simulink model "gap_generation_single_veh_state_machine"  (R2019a)
settings: Solver=VariableStepAuto  StartTime=0.0  StopTime=40  FixedStep=0.1  RelTol=1e-3
undefined symbols (not defined in the file): DiscIntNeverNeededParam
libraries: simulink x43, powerlib_meascontrol x5, autolibshared x5
(part 3 of 3)

== system gap_generation_single_veh_state_machine/Lo/ACC/Headway error ==
  xf : Inport
  vf : Inport  Port=2
  xl : Inport  Port=3
  lcFlag : Inport  Port=4
  Compare To Constant : simulink/Logic and Bit Operations/Compare To Constant  relop=<=  const=0  OutDataTypeStr=boolean
  Demux{,1..3} (4 alike) : Demux  Outputs=2
  Integrator : Integrator  InitialCondition=[h d0]
  Multiply : Product
  Mux : Mux  Inputs=2
  Mux1 : Mux  Inputs=2
  Product : Product
  Sum : Sum  Inputs=-+|
  Sum1 : Sum  Inputs=++|
  Sum2 : Sum  Inputs=+-|
  Sum3 : Sum  Inputs=|++
  Sum4 : Sum  Inputs=|+-
  Sum5 : Sum  Inputs=+-|
  Sum6 : Sum  Inputs=|++
  Switch : Switch  Criteria=u2 > Threshold
  Terminator : Terminator
  Terminator1 : Terminator
  d0 : Constant  Value=d0
  d0Lc : Constant  Value=d0Lc
  h : Constant  Value=h
  h scope : Scope  NumInputPorts=2
  hFilterGain : Gain  Gain=hFilterGain
  hLc : Constant  Value=hLc
  vLen : Constant  Value=lr+lf
  eh : Outport
  "gap " : Outport  Port=2
  unsafeFlag : Outport  Port=3
  wires:
  Demux3/2 -> Terminator1/1
  Demux2/2 -> Terminator/1
  Demux3/1 -> h scope/2
  Demux2/1 -> h scope/1
  Sum6/1 -> Sum5/2  "safe  gap"
  Demux1/2 -> Sum6/2  "gap at  standstill"
  Product/1 -> Sum6/1
  Demux1/1 -> Product/2  "time headway"
  Compare To Constant/1 -> unsafeFlag/1
  Sum5/1 -> Compare To Constant/1
  hFilterGain/1 -> Integrator/1
  Demux/2 -> Sum3/2  "gap at  standstill"
  Demux/1 -> Multiply/2  "time headway"
  Mux1/1 -> Switch/1
  d0Lc/1 -> Mux1/2
  hLc/1 -> Mux1/1
  Mux/1 -> Switch/3, Demux1/1  "min safe gap"
  d0/1 -> Mux/2
  Sum2/1 -> eh/1
  lcFlag/1 -> Switch/2
  Integrator/1 -> Demux/1, Sum4/2, Demux3/1
  Sum4/1 -> hFilterGain/1
  Switch/1 -> Sum4/1, Demux2/1
  h/1 -> Mux/1
  xl/1 -> Sum/2
  Sum1/1 -> Sum/1  "x (front bumber)"
  vf/1 -> Multiply/1, Product/1
  Sum3/1 -> Sum2/2  "desired  gap"
  xf/1 -> Sum1/2
  Sum/1 -> Sum2/1, "gap "/1, Sum5/1  "gap"
  Multiply/1 -> Sum3/1
  vLen/1 -> Sum1/1

== system gap_generation_single_veh_state_machine/Lo/ACC-v/Headway error ==
  xf : Inport
  vf : Inport  Port=2
  xl : Inport  Port=3
  lcFlag : Inport  Port=4
  Demux : Demux  Outputs=2
  Integrator : Integrator  InitialCondition=h
  Multiply : Product
  Mux : Mux  Inputs=2
  Mux1 : Mux  Inputs=2
  Sum : Sum  Inputs=-+|
  Sum1 : Sum  Inputs=++|
  Sum2 : Sum  Inputs=+-|
  Sum3 : Sum  Inputs=|++
  Sum4 : Sum  Inputs=|+-
  Switch : Switch  Criteria=u2 > Threshold
  d0 : Constant  Value=d0
  d0Lc : Constant  Value=d0Lc
  h : Constant  Value=h
  hFilterGain : Gain  Gain=hFilterGain
  hLc : Constant  Value=hLc
  vLen : Constant  Value=lr+lf
  eh : Outport
  "gap " : Outport  Port=2
  wires:
  Demux/2 -> Sum3/2  "gap at  standstill"
  Demux/1 -> Multiply/2  "time headway"
  Mux1/1 -> Switch/1
  d0Lc/1 -> Mux1/2
  hLc/1 -> Mux1/1
  Mux/1 -> Switch/3
  d0/1 -> Mux/2
  Sum2/1 -> eh/1
  lcFlag/1 -> Switch/2
  Integrator/1 -> Demux/1, Sum4/2
  Sum4/1 -> hFilterGain/1
  hFilterGain/1 -> Integrator/1
  Switch/1 -> Sum4/1
  h/1 -> Mux/1
  xl/1 -> Sum/2
  Sum1/1 -> Sum/1  "x (front bumber)"
  vf/1 -> Multiply/1
  Sum3/1 -> Sum2/2  "desired  gap"
  xf/1 -> Sum1/2
  Sum/1 -> Sum2/1, "gap "/1  "gap"
  Multiply/1 -> Sum3/1
  vLen/1 -> Sum1/1

== system gap_generation_single_veh_state_machine/Lo/ACC-v/Triggered Subsystem ==
  Trigger : TriggerPort  VariantControl=Variant
  Constant : Constant
  Out1 : Outport  InitialOutput=0
  wires:
  Constant/1 -> Out1/1

== system gap_generation_single_veh_state_machine/Lo/ACC-v/Triggered Subsystem1 ==
  Trigger : TriggerPort  VariantControl=Variant
  Constant : Constant  Value=0
  Out1 : Outport  InitialOutput=1
  wires:
  Constant/1 -> Out1/1

== system gap_generation_single_veh_state_machine/p1/ACC/Headway error ==
  xf : Inport
  vf : Inport  Port=2
  xl : Inport  Port=3
  lcFlag : Inport  Port=4
  Compare To Constant : simulink/Logic and Bit Operations/Compare To Constant  relop=<=  const=0  OutDataTypeStr=boolean
  Demux{,1..3} (4 alike) : Demux  Outputs=2
  Integrator : Integrator  InitialCondition=[h d0]
  Multiply : Product
  Mux : Mux  Inputs=2
  Mux1 : Mux  Inputs=2
  Product : Product
  Sum : Sum  Inputs=-+|
  Sum1 : Sum  Inputs=++|
  Sum2 : Sum  Inputs=+-|
  Sum3 : Sum  Inputs=|++
  Sum4 : Sum  Inputs=|+-
  Sum5 : Sum  Inputs=+-|
  Sum6 : Sum  Inputs=|++
  Switch : Switch  Criteria=u2 > Threshold
  Terminator : Terminator
  Terminator1 : Terminator
  d0 : Constant  Value=d0
  d0Lc : Constant  Value=d0Lc
  h : Constant  Value=h
  h scope : Scope  NumInputPorts=2
  hFilterGain : Gain  Gain=hFilterGain
  hLc : Constant  Value=hLc
  vLen : Constant  Value=lr+lf
  eh : Outport
  "gap " : Outport  Port=2
  unsafeFlag : Outport  Port=3
  wires:
  vLen/1 -> Sum1/1
  Multiply/1 -> Sum3/1
  Sum/1 -> Sum5/1, "gap "/1, Sum2/1  "gap"
  xf/1 -> Sum1/2
  Sum3/1 -> Sum2/2  "desired  gap"
  vf/1 -> Product/1, Multiply/1
  Sum1/1 -> Sum/1  "x (front bumber)"
  xl/1 -> Sum/2
  h/1 -> Mux/1
  Switch/1 -> Demux2/1, Sum4/1
  Sum4/1 -> hFilterGain/1
  Integrator/1 -> Demux3/1, Sum4/2, Demux/1
  lcFlag/1 -> Switch/2
  Sum2/1 -> eh/1
  d0/1 -> Mux/2
  Mux/1 -> Demux1/1, Switch/3  "min safe gap"
  hLc/1 -> Mux1/1
  d0Lc/1 -> Mux1/2
  Mux1/1 -> Switch/1
  Demux/1 -> Multiply/2  "time headway"
  Demux/2 -> Sum3/2  "gap at  standstill"
  hFilterGain/1 -> Integrator/1
  Sum5/1 -> Compare To Constant/1
  Compare To Constant/1 -> unsafeFlag/1
  Demux1/1 -> Product/2  "time headway"
  Product/1 -> Sum6/1
  Demux1/2 -> Sum6/2  "gap at  standstill"
  Sum6/1 -> Sum5/2  "safe  gap"
  Demux2/1 -> h scope/1
  Demux3/1 -> h scope/2
  Demux2/2 -> Terminator/1
  Demux3/2 -> Terminator1/1

== system gap_generation_single_veh_state_machine/p1/Chart/RegularVehFollowing.vehFollowing/ACC ==
  note: Vehicle following
  note: Switch logic (veh foll to vel control)
  note: Velocity control
  note: If there's no leader or the leader
      | is too far away, use velocity control
  currentStates : Inport  OutDataTypeStr=Bus: vehStates
  leaderStates : Inport  Port=2  OutDataTypeStr=Bus: vehStates  PortDimensions=4
  lcFlag : Inport  Port=3
  ACC outputs : Scope  NumInputPorts=3
  AND : Logic  IconShape=distinctive  AllPortsSameDT=off  OutDataTypeStr=boolean
  Anti-windup gain : Gain  Gain=sqrt(Ki/Kd)
  Bus Selector : BusSelector  OutputSignals=X,Xdot,u
  Bus Selector1 : BusSelector  OutputSignals=X,Xdot
  Compare To Constant : simulink/Logic and Bit Operations/Compare To Constant  relop=<  const=2*maxHeadwayError  OutDataTypeStr=boolean
  Compare To Constant1 : simulink/Logic and Bit Operations/Compare To Constant  relop=>  const=0  OutDataTypeStr=boolean
  Discrete-Time Integrator : DiscreteIntegrator  SampleTime=-1  ICPrevOutput=DiscIntNeverNeededParam  ICPrevScaledInput=DiscIntNeverNeededParam
  Discrete-Time Integrator1 : DiscreteIntegrator  ExternalReset=either  SampleTime=-1  ICPrevOutput=DiscIntNeverNeededParam  ICPrevScaledInput=DiscIntNeverNeededParam
  Discrete-Time Integrator2 : DiscreteIntegrator  IntegratorMethod=Integration: Trapezoidal  InitialCondition=vx0  SampleTime=-1  ICPrevOutput=DiscIntNeverNeededParam  ICPrevScaledInput=DiscIntNeverNeededParam
  Gain3 : Gain  Gain=velFilterGain
  Headway error : Subsystem
  Kd : Gain  Gain=Kd
  Ki : Gain  Gain=Ki
  Kp : Gain  Gain=Kp
  Mux : Mux  Inputs=2
  Saturation : Saturate  UpperLimit=maxAcceleration  LowerLimit=minAcceleration
  Saturation1 : Saturate  UpperLimit=maxHeadwayError  LowerLimit=minHeadwayError
  Scope : Scope  NumInputPorts=3
  Signal Specification{,1..4} (5 alike) : SignalSpecification  Dimensions=1
  Sum : Sum  Inputs=-+|
  Sum1 : Sum  Inputs=+++
  Sum2 : Sum  Inputs=|+-
  Sum3 : Sum
  Sum4 : Sum  Inputs=+-
  Sum5 : Sum  Inputs=-+|
  Switch : Switch  Criteria=u2 > Threshold
  Terminator : Terminator
  safe saturation : Saturate  UpperLimit=maxComfAccel  LowerLimit=minComfAccel
  velKi : Gain  Gain=velKi
  velKp : Gain  Gain=velKp
  u : Outport
  errors : Outport  Port=2  PortDimensions=2
  gap : Outport  Port=3
  wires:
  Headway error/1(eh) -> Saturation1/1, Mux/1, Compare To Constant/1
  Bus Selector/2 -> Headway error/2(vf), Sum/1  "<Xdot>"
  Kd/1 -> Scope/3, Sum1/3
  Kp/1 -> Signal Specification4/1
  Gain3/1 -> Saturation/1
  Saturation/1 -> Discrete-Time Integrator2/1
  Bus Selector1/2 -> Sum2/1  "<Xdot>"
  Sum2/1 -> Gain3/1
  Saturation1/1 -> Kp/1, Ki/1
  Headway error/2("gap ") -> gap/1
  Discrete-Time Integrator/1 -> velKi/1
  velKi/1 -> Sum3/2
  Switch/1 -> Sum4/1, safe saturation/1  "u"
  Sum1/1 -> Signal Specification3/1
  Sum3/1 -> ACC outputs/3, Switch/3
  Sum/1 -> Mux/2, Kd/1, Discrete-Time Integrator/1, velKp/1
  Mux/1 -> errors/1
  Sum5/1 -> Discrete-Time Integrator1/1
  velKp/1 -> Sum3/1
  Ki/1 -> Sum5/2
  Discrete-Time Integrator1/1 -> Sum1/1, Scope/1
  Anti-windup gain/1 -> Sum5/1
  AND/1 -> Discrete-Time Integrator1/2, Switch/2, ACC outputs/2
  Compare To Constant/1 -> Signal Specification2/1
  Compare To Constant1/1 -> AND/1
  currentStates/1 -> Bus Selector/1
  Bus Selector/1 -> Headway error/1(xf)  "<X>"
  leaderStates/1 -> Bus Selector1/1
  Bus Selector1/1 -> Compare To Constant1/1, Headway error/3(xl)  "<X>"
  Bus Selector/3 -> [realInput]  "<u>"
  [realInput] -> Sum4/2
  safe saturation/1 -> u/1  "sat(u)"
  lcFlag/1 -> Terminator/1
  Discrete-Time Integrator2/1 -> Signal Specification/1, Sum/2
  Sum4/1 -> Signal Specification1/1
  Signal Specification/1 -> Sum2/2
  Signal Specification1/1 -> Anti-windup gain/1
  Signal Specification2/1 -> AND/2
  Signal Specification3/1 -> Switch/1, ACC outputs/1
  Signal Specification4/1 -> Scope/2, Sum1/2

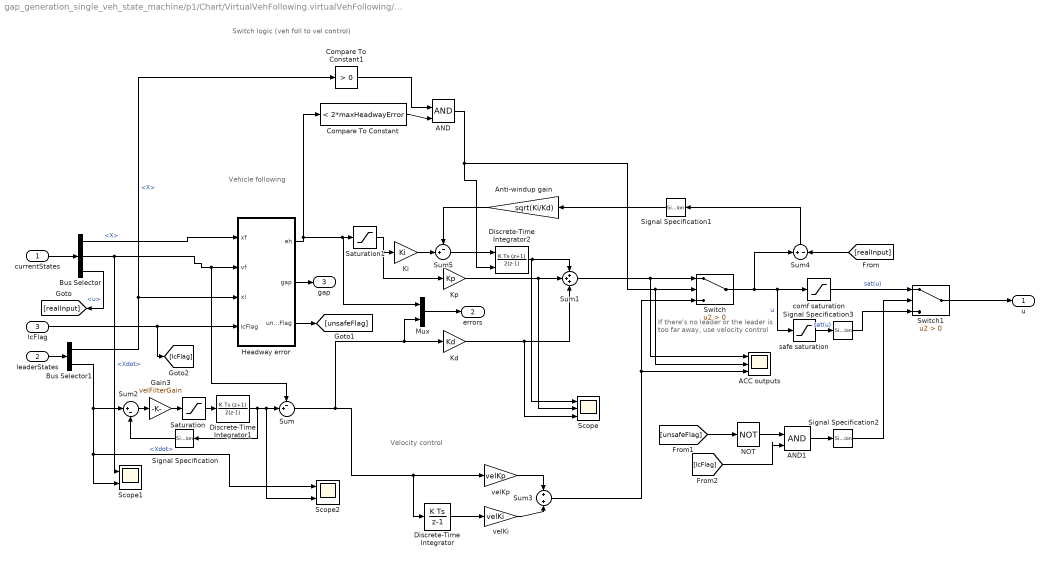
== system gap_generation_single_veh_state_machine/p1/Chart/VirtualVehFollowing.virtualVehFollowing/ACC ==
  note: Vehicle following
  note: Switch logic (veh foll to vel control)
  note: Velocity control
  note: If there's no leader or the leader
      | is too far away, use velocity control
  currentStates : Inport  OutDataTypeStr=Bus: vehStates
  leaderStates : Inport  Port=2  OutDataTypeStr=Bus: vehStates
  lcFlag : Inport  Port=3
  ACC outputs : Scope  NumInputPorts=3
  AND : Logic  IconShape=distinctive  AllPortsSameDT=off  OutDataTypeStr=boolean
  AND1 : Logic  IconShape=distinctive  AllPortsSameDT=off  OutDataTypeStr=boolean
  Anti-windup gain : Gain  Gain=sqrt(Ki/Kd)
  Bus Selector : BusSelector  OutputSignals=X,Xdot,u
  Bus Selector1 : BusSelector  OutputSignals=X,Xdot
  Compare To Constant : simulink/Logic and Bit Operations/Compare To Constant  relop=<  const=2*maxHeadwayError  OutDataTypeStr=boolean
  Compare To Constant1 : simulink/Logic and Bit Operations/Compare To Constant  relop=>  const=0  OutDataTypeStr=boolean
  Discrete-Time Integrator : DiscreteIntegrator  SampleTime=-1  ICPrevOutput=DiscIntNeverNeededParam  ICPrevScaledInput=DiscIntNeverNeededParam
  Discrete-Time Integrator1 : DiscreteIntegrator  IntegratorMethod=Integration: Trapezoidal  InitialCondition=vx0  SampleTime=-1  ICPrevOutput=DiscIntNeverNeededParam  ICPrevScaledInput=DiscIntNeverNeededParam
  Discrete-Time Integrator2 : DiscreteIntegrator  IntegratorMethod=Integration: Trapezoidal  ExternalReset=either  SampleTime=-1  ICPrevOutput=DiscIntNeverNeededParam  ICPrevScaledInput=DiscIntNeverNeededParam
  Gain3 : Gain  Gain=velFilterGain
  Headway error : Subsystem
  Kd : Gain  Gain=Kd
  Ki : Gain  Gain=Ki
  Kp : Gain  Gain=Kp
  Mux : Mux  Inputs=2
  NOT : Logic  Operator=NOT  IconShape=distinctive  AllPortsSameDT=off  OutDataTypeStr=boolean
  Saturation : Saturate  UpperLimit=maxAcceleration  LowerLimit=minAcceleration
  Saturation1 : Saturate  UpperLimit=maxHeadwayError  LowerLimit=minHeadwayError
  Scope : Scope  NumInputPorts=3
  Scope1 : Scope  NumInputPorts=2
  Scope2 : Scope  NumInputPorts=2
  Signal Specification{,1..3} (4 alike) : SignalSpecification  Dimensions=1
  Sum : Sum  Inputs=-+|
  Sum1 : Sum  Inputs=+++
  Sum2 : Sum  Inputs=|+-
  Sum3 : Sum
  Sum4 : Sum  Inputs=+-
  Sum5 : Sum  Inputs=-+|
  Switch : Switch  Criteria=u2 > Threshold
  Switch1 : Switch  Criteria=u2 > Threshold
  comf saturation : Saturate  UpperLimit=2  LowerLimit=-2
  safe saturation : Saturate  UpperLimit=maxComfAccel  LowerLimit=minComfAccel
  velKi : Gain  Gain=velKi
  velKp : Gain  Gain=velKp
  u : Outport  PortDimensions=1
  errors : Outport  Port=2  PortDimensions=2
  gap : Outport  Port=3  PortDimensions=1
  wires:
  Headway error/1(eh) -> Saturation1/1, Mux/1, Compare To Constant/1
  Bus Selector/2 -> Scope1/1, Headway error/2(vf), Sum/1  "<Xdot>"
  Kd/1 -> Scope/3, Sum1/3
  Kp/1 -> Scope/2, Sum1/2
  Gain3/1 -> Saturation/1
  Saturation/1 -> Discrete-Time Integrator1/1
  Bus Selector1/2 -> Scope2/1, Scope1/2, Sum2/1  "<Xdot>"
  Sum2/1 -> Gain3/1
  Saturation1/1 -> Kp/1, Ki/1
  Headway error/2("gap ") -> gap/1
  Discrete-Time Integrator/1 -> velKi/1
  velKi/1 -> Sum3/2
  Switch/1 -> Sum4/1, safe saturation/1, comf saturation/1  "u"
  Sum1/1 -> Switch/1, ACC outputs/1
  Sum3/1 -> ACC outputs/3, Switch/3
  Sum/1 -> Mux/2, Kd/1, Discrete-Time Integrator/1, velKp/1
  Mux/1 -> errors/1
  Sum5/1 -> Discrete-Time Integrator2/1
  velKp/1 -> Sum3/1
  Ki/1 -> Sum5/2
  Discrete-Time Integrator2/1 -> Scope/1, Sum1/1
  Anti-windup gain/1 -> Sum5/1
  AND/1 -> Discrete-Time Integrator2/2, Switch/2, ACC outputs/2
  Compare To Constant/1 -> AND/2
  Compare To Constant1/1 -> AND/1
  lcFlag/1 -> [lcFlag], Headway error/4(lcFlag)
  currentStates/1 -> Bus Selector/1
  Bus Selector/1 -> Headway error/1(xf)  "<X>"
  leaderStates/1 -> Bus Selector1/1
  Bus Selector1/1 -> Compare To Constant1/1, Headway error/3(xl)  "<X>"
  Bus Selector/3 -> [realInput]  "<u>"
  [realInput] -> Sum4/2
  Headway error/3(unsafeFlag) -> [unsafeFlag]
  [unsafeFlag] -> NOT/1
  NOT/1 -> AND1/1
  [lcFlag] -> AND1/2
  AND1/1 -> Signal Specification2/1
  safe saturation/1 -> Signal Specification3/1  "sat(u)"
  Switch1/1 -> u/1
  comf saturation/1 -> Switch1/1  "sat(u)"
  Discrete-Time Integrator1/1 -> Signal Specification/1, Scope2/2, Sum/2
  Sum4/1 -> Signal Specification1/1
  Signal Specification/1 -> Sum2/2
  Signal Specification1/1 -> Anti-windup gain/1
  Signal Specification2/1 -> Switch1/2
  Signal Specification3/1 -> Switch1/3

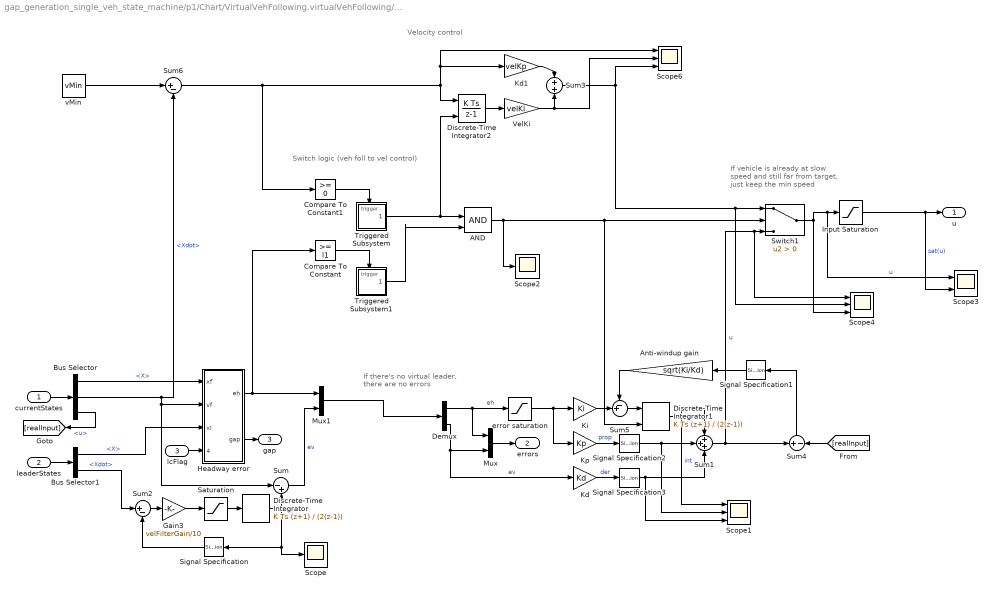
== system gap_generation_single_veh_state_machine/p1/Chart/VirtualVehFollowing.virtualVehFollowing/ACC-v ==
  note: If vehicle is already at slow
      | speed and still far from target,
      | just keep the min speed
  note: If there's no virtual leader,
      | there are no errors
  note: Switch logic (veh foll to vel control)
  note: Velocity control
  currentStates : Inport
  leaderStates : Inport  Port=2
  lcFlag : Inport  Port=3
  AND : Logic  IconShape=distinctive  AllPortsSameDT=off  OutDataTypeStr=boolean
  Anti-windup gain : Gain  Gain=sqrt(Ki/Kd)
  Bus Selector : BusSelector  OutputSignals=X,Xdot,u
  Bus Selector1 : BusSelector  OutputSignals=X,Xdot
  Compare To Constant : simulink/Logic and Bit Operations/Compare To Constant  relop=>=  const=l1  OutDataTypeStr=boolean
  Compare To Constant1 : simulink/Logic and Bit Operations/Compare To Constant  relop=>=  const=0  OutDataTypeStr=boolean
  Demux : Demux  Outputs=2
  Discrete-Time Integrator : DiscreteIntegrator  IntegratorMethod=Integration: Trapezoidal  InitialCondition=vx0  SampleTime=-1  ICPrevOutput=DiscIntNeverNeededParam  ICPrevScaledInput=DiscIntNeverNeededParam
  Discrete-Time Integrator1 : DiscreteIntegrator  IntegratorMethod=Integration: Trapezoidal  ExternalReset=falling  SampleTime=-1  ICPrevOutput=DiscIntNeverNeededParam  ICPrevScaledInput=DiscIntNeverNeededParam
  Discrete-Time Integrator2 : DiscreteIntegrator  ExternalReset=rising  SampleTime=-1  ICPrevOutput=DiscIntNeverNeededParam  ICPrevScaledInput=DiscIntNeverNeededParam
  Gain3 : Gain  Gain=velFilterGain/10
  Headway error : Subsystem
  Input Saturation : Saturate  UpperLimit=maxComfAccel  LowerLimit=minComfAccel
  Kd : Gain  Gain=Kd
  Kd1 : Gain  Gain=velKp
  Ki : Gain  Gain=Ki
  Kp : Gain  Gain=Kp
  Mux : Mux  Inputs=2
  Mux1 : Mux  Inputs=2
  Saturation : Saturate  UpperLimit=maxAcceleration  LowerLimit=minAcceleration
  Scope : Scope
  Scope1 : Scope  NumInputPorts=3
  Scope2 : Scope
  Scope3 : Scope  NumInputPorts=2
  Scope4 : Scope  NumInputPorts=3
  Scope6 : Scope  NumInputPorts=3
  Signal Specification{,1..3} (4 alike) : SignalSpecification  Dimensions=1
  Sum : Sum  Inputs=|-+
  Sum1 : Sum  Inputs=+++
  Sum2 : Sum  Inputs=|+-
  Sum3 : Sum
  Sum4 : Sum  Inputs=+-
  Sum5 : Sum  Inputs=-+|
  Sum6 : Sum  Inputs=|+-
  Switch1 : Switch  Criteria=u2 > Threshold
  Triggered Subsystem : Subsystem  TreatAsAtomicUnit=on
  Triggered Subsystem1 : Subsystem  TreatAsAtomicUnit=on
  VelKi : Gain  Gain=velKi
  error saturation : Saturate  UpperLimit=maxHeadwayError  LowerLimit=minHeadwayError/10
  vMin : Constant  Value=vMin
  u : Outport  PortDimensions=1  OutputWhenDisabled=reset  InitialOutput=0
  errors : Outport  Port=2  OutputWhenDisabled=reset  InitialOutput=[0, 0]
  gap : Outport  Port=3  OutputWhenDisabled=reset  InitialOutput=[0]
  wires:
  Kd/1 -> Signal Specification3/1  "der"
  Switch1/1 -> Scope3/1, Input Saturation/1, Scope4/3  "u"
  Headway error/1(eh) -> Mux1/1, Compare To Constant/1
  vMin/1 -> Sum6/1
  Anti-windup gain/1 -> Sum5/1
  Saturation/1 -> Discrete-Time Integrator/1
  Sum/1 -> Mux1/2  "ev"
  Demux/2 -> Mux/2, Kd/1  "ev"
  Discrete-Time Integrator1/1 -> Sum1/1, Scope1/1  "int"
  Mux1/1 -> Demux/1
  Discrete-Time Integrator/1 -> Scope/1, Signal Specification/1, Sum/2
  Compare To Constant/1 -> Triggered Subsystem1/Trigger
  Sum6/1 -> Discrete-Time Integrator2/1, Scope6/1, Kd1/1, Compare To Constant1/1
  Sum3/1 -> Scope6/3, Scope4/2, Switch1/1
  Bus Selector/2 -> Sum6/2, Headway error/2(vf), Sum/1  "<Xdot>"
  Gain3/1 -> Saturation/1
  Sum4/1 -> Signal Specification1/1
  Demux/1 -> error saturation/1, Mux/1  "eh"
  Kd1/1 -> Sum3/1
  Headway error/2("gap ") -> gap/1
  Discrete-Time Integrator2/1 -> VelKi/1
  [realInput] -> Sum4/2
  Ki/1 -> Sum5/2
  Input Saturation/1 -> Scope3/2, u/1  "sat(u)"
  Sum1/1 -> Scope4/1, Switch1/3, Sum4/1  "u"
  VelKi/1 -> Scope6/2, Sum3/2
  currentStates/1 -> Bus Selector/1
  Sum5/1 -> Discrete-Time Integrator1/1
  Bus Selector1/1 -> Headway error/3(xl)  "<X>"
  error saturation/1 -> Kp/1, Ki/1
  Mux/1 -> errors/1
  Bus Selector1/2 -> Sum2/1  "<Xdot>"
  Bus Selector/1 -> Headway error/1(xf)  "<X>"
  Triggered Subsystem/1(Out1) -> Discrete-Time Integrator2/2, AND/1
  Sum2/1 -> Gain3/1
  leaderStates/1 -> Bus Selector1/1
  lcFlag/1 -> Headway error/4(lcFlag)
  Bus Selector/3 -> [realInput]  "<u>"
  Triggered Subsystem1/1(Out1) -> AND/2
  Compare To Constant1/1 -> Triggered Subsystem/Trigger
  Kp/1 -> Signal Specification2/1  "prop"
  AND/1 -> Discrete-Time Integrator1/2, Switch1/2, Scope2/1
  Signal Specification/1 -> Sum2/2
  Signal Specification1/1 -> Anti-windup gain/1
  Signal Specification2/1 -> Scope1/2, Sum1/2
  Signal Specification3/1 -> Scope1/3, Sum1/3

== system gap_generation_single_veh_state_machine/p1/Enabled Subsystem/Headway error ==
  xf : Inport
  vf : Inport  Port=2
  xl : Inport  Port=3
  lcFlag : Inport  Port=4
  Demux : Demux  Outputs=2
  Integrator : Integrator  InitialCondition=h
  Multiply : Product
  Mux : Mux  Inputs=2
  Mux1 : Mux  Inputs=2
  Sum : Sum  Inputs=-+|
  Sum1 : Sum  Inputs=++|
  Sum2 : Sum  Inputs=+-|
  Sum3 : Sum  Inputs=|++
  Sum4 : Sum  Inputs=|+-
  Switch : Switch  Criteria=u2 > Threshold
  d0 : Constant  Value=d0
  d0Lc : Constant  Value=d0Lc
  h : Constant  Value=h
  hFilterGain : Gain  Gain=hFilterGain
  hLc : Constant  Value=hLc
  vLen : Constant  Value=lr+lf
  eh : Outport
  "gap " : Outport  Port=2
  wires:
  vLen/1 -> Sum1/1
  Multiply/1 -> Sum3/1
  Sum/1 -> "gap "/1, Sum2/1  "gap"
  xf/1 -> Sum1/2
  Sum3/1 -> Sum2/2  "desired  gap"
  vf/1 -> Multiply/1
  Sum1/1 -> Sum/1  "x (front bumber)"
  xl/1 -> Sum/2
  h/1 -> Mux/1
  Switch/1 -> Sum4/1
  hFilterGain/1 -> Integrator/1
  Sum4/1 -> hFilterGain/1
  Integrator/1 -> Sum4/2, Demux/1
  lcFlag/1 -> Switch/2
  Sum2/1 -> eh/1
  d0/1 -> Mux/2
  Mux/1 -> Switch/3
  hLc/1 -> Mux1/1
  d0Lc/1 -> Mux1/2
  Mux1/1 -> Switch/1
  Demux/1 -> Multiply/2  "time headway"
  Demux/2 -> Sum3/2  "gap at  standstill"

== system gap_generation_single_veh_state_machine/p1/Enabled Subsystem/Triggered Subsystem ==
  Trigger : TriggerPort  VariantControl=Variant
  Constant : Constant
  Out1 : Outport  InitialOutput=0
  wires:
  Constant/1 -> Out1/1

== system gap_generation_single_veh_state_machine/p1/Enabled Subsystem/Triggered Subsystem1 ==
  Trigger : TriggerPort  VariantControl=Variant
  Constant : Constant  Value=0
  Out1 : Outport  InitialOutput=1
  wires:
  Constant/1 -> Out1/1

== system gap_generation_single_veh_state_machine/p1/Chart/RegularVehFollowing.vehFollowing/ACC/Headway error ==
  xf : Inport
  vf : Inport  Port=2
  xl : Inport  Port=3
  Multiply : Product
  Sum : Sum  Inputs=-+|
  Sum1 : Sum  Inputs=++|
  Sum2 : Sum  Inputs=+-|
  Sum3 : Sum  Inputs=|++
  d0 : Constant  Value=d0
  h : Constant  Value=h
  vLen : Constant  Value=lr+lf
  eh : Outport  PortDimensions=1
  "gap " : Outport  Port=2  PortDimensions=1
  wires:
  vLen/1 -> Sum1/1
  Multiply/1 -> Sum3/1
  Sum/1 -> "gap "/1, Sum2/1  "gap"
  xf/1 -> Sum1/2
  Sum3/1 -> Sum2/2  "desired  gap"
  vf/1 -> Multiply/1
  Sum1/1 -> Sum/1  "x (front bumber)"
  xl/1 -> Sum/2
  Sum2/1 -> eh/1
  h/1 -> Multiply/2  "time headway"
  d0/1 -> Sum3/2  "gap at  standstill"

== system gap_generation_single_veh_state_machine/p1/Chart/VirtualVehFollowing.virtualVehFollowing/ACC/Headway error ==
  xf : Inport
  vf : Inport  Port=2
  xl : Inport  Port=3
  lcFlag : Inport  Port=4
  Compare To Constant : simulink/Logic and Bit Operations/Compare To Constant  relop=<=  const=0  OutDataTypeStr=boolean
  Demux{,1..3} (4 alike) : Demux  Outputs=2
  Discrete-Time Integrator : DiscreteIntegrator  IntegratorMethod=Integration: Trapezoidal  InitialCondition=[h d0]  SampleTime=-1  ICPrevOutput=DiscIntNeverNeededParam  ICPrevScaledInput=DiscIntNeverNeededParam
  Multiply : Product
  Mux : Mux  Inputs=2
  Mux1 : Mux  Inputs=2
  Product : Product
  Signal Specification : SignalSpecification  Dimensions=2
  Signal Specification1 : SignalSpecification  Dimensions=1
  Signal Specification2 : SignalSpecification  Dimensions=1
  Sum : Sum  Inputs=-+|
  Sum1 : Sum  Inputs=++|
  Sum2 : Sum  Inputs=+-|
  Sum3 : Sum  Inputs=|++
  Sum4 : Sum  Inputs=|+-
  Sum5 : Sum  Inputs=+-|
  Sum6 : Sum  Inputs=|++
  Switch : Switch  Criteria=u2 > Threshold
  Terminator : Terminator
  Terminator1 : Terminator
  d0 : Constant  Value=d0
  d0Lc : Constant  Value=d0Lc
  h : Constant  Value=h
  h scope : Scope  NumInputPorts=2
  hFilterGain : Gain  Gain=hFilterGain
  hLc : Constant  Value=hLc
  vLen : Constant  Value=lr+lf
  eh : Outport
  "gap " : Outport  Port=2
  unsafeFlag : Outport  Port=3  PortDimensions=1
  wires:
  vLen/1 -> Sum1/1
  Multiply/1 -> Sum3/1
  Sum/1 -> Sum5/1, "gap "/1, Sum2/1  "gap"
  xf/1 -> Sum1/2
  Sum3/1 -> Sum2/2  "desired  gap"
  vf/1 -> Signal Specification2/1
  Sum1/1 -> Signal Specification1/1  "x (front bumber)"
  xl/1 -> Sum/2
  h/1 -> Mux/1
  Switch/1 -> Demux2/1, Sum4/1
  Sum4/1 -> hFilterGain/1
  Discrete-Time Integrator/1 -> Demux3/1, Signal Specification/1, Demux/1
  lcFlag/1 -> Switch/2
  Sum2/1 -> eh/1
  d0/1 -> Mux/2
  Mux/1 -> Demux1/1, Switch/3  "min safe gap"
  hLc/1 -> Mux1/1
  d0Lc/1 -> Mux1/2
  Mux1/1 -> Switch/1
  Demux/1 -> Multiply/2  "time headway"
  Demux/2 -> Sum3/2  "gap at  standstill"
  hFilterGain/1 -> Discrete-Time Integrator/1
  Sum5/1 -> Compare To Constant/1
  Compare To Constant/1 -> unsafeFlag/1
  Demux1/1 -> Product/2  "time headway"
  Product/1 -> Sum6/1
  Demux1/2 -> Sum6/2  "gap at  standstill"
  Sum6/1 -> Sum5/2  "safe  gap"
  Demux2/1 -> h scope/1
  Demux3/1 -> h scope/2
  Demux2/2 -> Terminator/1
  Demux3/2 -> Terminator1/1
  Signal Specification/1 -> Sum4/2
  Signal Specification1/1 -> Sum/1
  Signal Specification2/1 -> Product/1, Multiply/1

== system gap_generation_single_veh_state_machine/p1/Chart/VirtualVehFollowing.virtualVehFollowing/ACC-v/Headway error ==
  xf : Inport
  vf : Inport  Port=2
  xl : Inport  Port=3
  lcFlag : Inport  Port=4
  Demux : Demux  Outputs=2
  Discrete-Time Integrator : DiscreteIntegrator  IntegratorMethod=Integration: Trapezoidal  InitialCondition=h  SampleTime=-1  ICPrevOutput=DiscIntNeverNeededParam  ICPrevScaledInput=DiscIntNeverNeededParam
  Multiply : Product
  Mux : Mux  Inputs=2
  Mux1 : Mux  Inputs=2
  Signal Specification : SignalSpecification  Dimensions=2
  Sum : Sum  Inputs=-+|
  Sum1 : Sum  Inputs=++|
  Sum2 : Sum  Inputs=+-|
  Sum3 : Sum  Inputs=|++
  Sum4 : Sum  Inputs=|+-
  Switch : Switch  Criteria=u2 > Threshold
  d0 : Constant  Value=d0
  d0Lc : Constant  Value=d0Lc
  h : Constant  Value=h
  hFilterGain : Gain  Gain=hFilterGain
  hLc : Constant  Value=hLc
  vLen : Constant  Value=lr+lf
  eh : Outport
  "gap " : Outport  Port=2
  wires:
  vLen/1 -> Sum1/1
  Multiply/1 -> Sum3/1
  Sum/1 -> "gap "/1, Sum2/1  "gap"
  xf/1 -> Sum1/2
  Sum3/1 -> Sum2/2  "desired  gap"
  vf/1 -> Multiply/1
  Sum1/1 -> Sum/1  "x (front bumber)"
  xl/1 -> Sum/2
  h/1 -> Mux/1
  Switch/1 -> Sum4/1
  hFilterGain/1 -> Discrete-Time Integrator/1
  Sum4/1 -> hFilterGain/1
  Discrete-Time Integrator/1 -> Demux/1, Signal Specification/1
  lcFlag/1 -> Switch/2
  Sum2/1 -> eh/1
  d0/1 -> Mux/2
  Mux/1 -> Switch/3
  hLc/1 -> Mux1/1
  d0Lc/1 -> Mux1/2
  Mux1/1 -> Switch/1
  Demux/1 -> Multiply/2  "time headway"
  Demux/2 -> Sum3/2  "gap at  standstill"
  Signal Specification/1 -> Sum4/2

== system gap_generation_single_veh_state_machine/p1/Chart/VirtualVehFollowing.virtualVehFollowing/ACC-v/Triggered Subsystem ==
  Trigger : TriggerPort  VariantControl=Variant
  Constant : Constant
  Out1 : Outport  InitialOutput=0
  wires:
  Constant/1 -> Out1/1

== system gap_generation_single_veh_state_machine/p1/Chart/VirtualVehFollowing.virtualVehFollowing/ACC-v/Triggered Subsystem1 ==
  Trigger : TriggerPort  VariantControl=Variant
  Constant : Constant  Value=0
  Out1 : Outport  InitialOutput=1
  wires:
  Constant/1 -> Out1/1

== stateflow chart gap_generation_single_veh_state_machine/p1/Chart ==
  state RegularVehFollowing
    entry:
    disp('in here')
    during:
    [u, eh, ev, gap] = vehFollowing(currentStates, leaderStates, lcFlag);
    state [u,eh,ev,gap] = vehFollowing(currentStates,leaderStates,lcFlag) [function]
  state VirtualVehFollowing
    during:
    [u, eh,ev, gap] = virtualVehFollowing(currentStates,virtualLeaderStates,lcFlag);
    state [u,eh,ev,gap] = virtualVehFollowing(currentStates,leaderStates,lcFlag) [function]
  (default) -> RegularVehFollowing
  RegularVehFollowing -> VirtualVehFollowing : [virtualFollowing==1]
  data: currentStates function_input Bus: vehStates size=1; leaderStates function_input Bus: vehStates size=1; lcFlag function_input double size=1; u function_output size=1; eh function_output size=1; ev function_output size=1; gap function_output size=1; currentStates function_input Bus: vehStates size=1; leaderStates function_input Bus: vehStates size=1; u function_output size=1; eh function_output size=1; ev function_output size=1; lcFlag function_input double size=1; gap function_output size=1; currentStates input; leaderStates input; lcFlag input; u output size=1; eh output size=1; ev output size=1; virtualFollowing input; virtualLeaderStates input; gap output size=1
